simulink model "s4dot2_33variantsubsystem"  (R2023b)
settings: Solver=VariableStepAuto  StartTime=0.0  StopTime=10.0  RelTol=1e-3
model workspace (MAT data in the model file):
  variant = 1
settings Model: Creator=lxj  LastModifiedBy=lxj

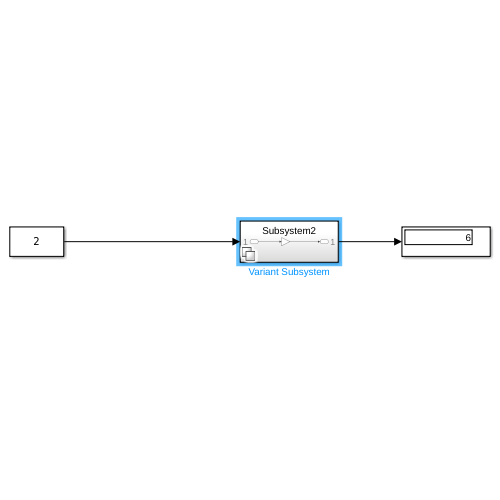
[thumbnail: Simulink's stored preview of the top-level diagram]
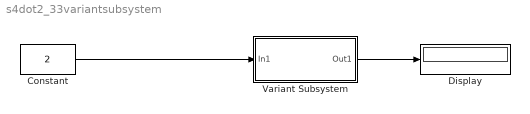
== system s4dot2_33variantsubsystem ==
  Constant : Constant  Value=2
  Display : Display
  Variant Subsystem : Subsystem  Variant=on
  wires:
  Constant/1 -> Variant Subsystem/1(In1)
  Variant Subsystem/1(Out1) -> Display/1

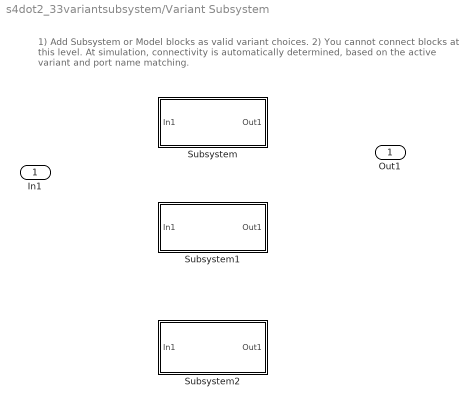
== system s4dot2_33variantsubsystem/Variant Subsystem ==
  note: 1) Add Subsystem or Model blocks as valid variant choices.
      | 2) You cannot connect blocks at this level. At simulation, connectivity is automatically
      | determined, based on the active variant and port name matching.
  In1 : Inport
  Subsystem : Subsystem  VariantControl=opt==1
  Subsystem1 : Subsystem  VariantControl=opt==2
  Subsystem2 : Subsystem  VariantControl=opt==3
  Out1 : Outport

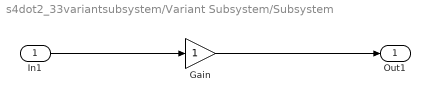
== system s4dot2_33variantsubsystem/Variant Subsystem/Subsystem ==
  In1 : Inport
  Gain : Gain
  Out1 : Outport
  wires:
  In1/1 -> Gain/1
  Gain/1 -> Out1/1

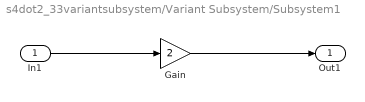
== system s4dot2_33variantsubsystem/Variant Subsystem/Subsystem1 ==
  In1 : Inport
  Gain : Gain  Gain=2
  Out1 : Outport
  wires:
  In1/1 -> Gain/1
  Gain/1 -> Out1/1

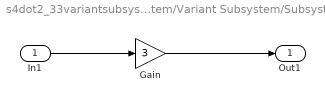
== system s4dot2_33variantsubsystem/Variant Subsystem/Subsystem2 ==
  In1 : Inport
  Gain : Gain  Gain=3
  Out1 : Outport
  wires:
  In1/1 -> Gain/1
  Gain/1 -> Out1/1
